simulink model "sampleModel145"  (R2021b)
settings: Solver=VariableStepAuto  StartTime=0.0  StopTime=10.0  RelTol=1e-3
libraries: simulink x1
settings Model: Creator=user  LastModifiedBy=user

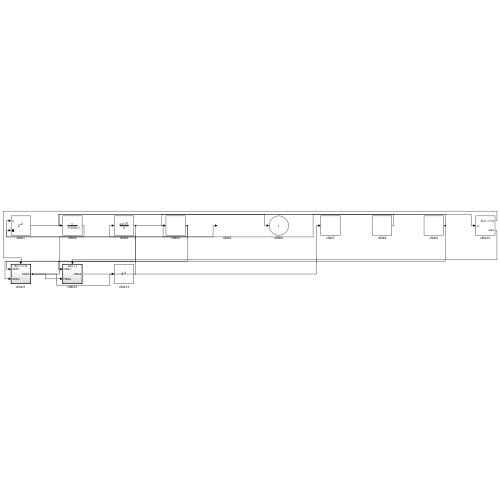
[thumbnail: Simulink's stored preview of the top-level diagram]
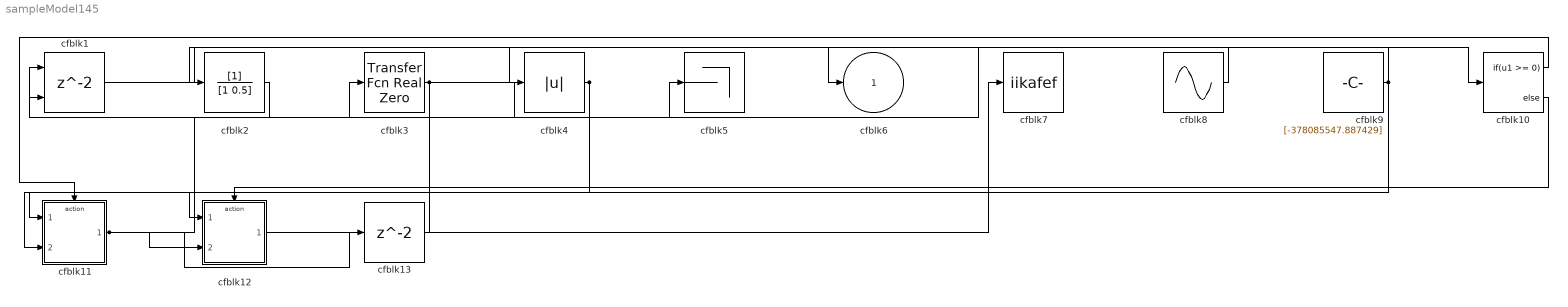
== system sampleModel145 ==
  cfblk1 : Delay  ShowEnablePort=on  SampleTime=1
      settings: InputPortMap=u0,e6
  cfblk10 : If  IfExpression=u1 >= 0  SampleTime=1
  cfblk11 : Subsystem  TreatAsAtomicUnit=on
  cfblk12 : Subsystem  TreatAsAtomicUnit=on
  cfblk13 : Delay  SampleTime=1
  cfblk2 : DiscreteFilter  SampleTime=1
  cfblk3 : simulink/Discrete/Transfer Fcn Real Zero  ZeroZ=0.75  ICPrevInput=0.0  DoSatur=off
      settings: SourceProductBaseCode=SL
  cfblk4 : Abs
  cfblk5 : Terminator
  cfblk7 : ToWorkspace  VariableName=iikafef  SaveFormat=Timeseries  SampleTime=-1
  cfblk8 : Sin  Amplitude=[-440683838.246815]  Bias=[450230892.144904]  SampleTime=0
  cfblk9 : Constant  Value=[-378085547.887429]  SampleTime=1
  cfblk6 : Outport
  wires:
  cfblk12/1(cfblk2) -> cfblk7/1
  cfblk1/1 -> cfblk6/1
  cfblk3/1 -> cfblk10/1, cfblk12/1(cfblk1)
  cfblk2/1 -> cfblk1/1
  cfblk11/1(cfblk2) -> cfblk5/1, cfblk12/2(cfblk4), cfblk13/1
  cfblk4/1 -> cfblk1/2, cfblk11/2(cfblk4)
  cfblk8/1 -> cfblk4/1
  cfblk9/1 -> cfblk2/1, cfblk11/1(cfblk1)
  cfblk10/1 -> cfblk11/Action
  cfblk10/2 -> cfblk12/Action
  cfblk13/1 -> cfblk3/1

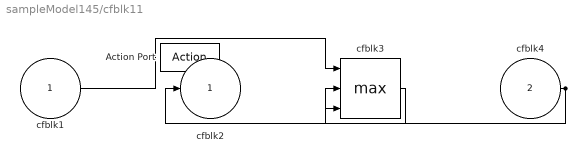
== system sampleModel145/cfblk11 ==
  cfblk1 : Inport
  cfblk4 : Inport  Port=2
  Action Port : ActionPort  ActionPortLabel=if(u1 >= 0)
  cfblk3 : MinMax  Function=max  Inputs=3
  cfblk2 : Outport
  wires:
  cfblk3/1 -> cfblk2/1
  cfblk1/1 -> cfblk3/1
  cfblk4/1 -> cfblk3/2, cfblk3/3

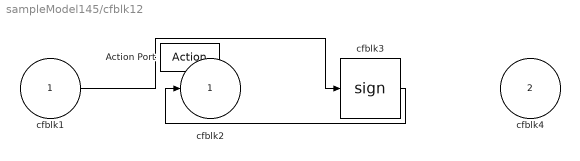
== system sampleModel145/cfblk12 ==
  cfblk1 : Inport
  cfblk4 : Inport  Port=2
  Action Port : ActionPort  ActionPortLabel=else
  cfblk3 : Signum
  cfblk2 : Outport
  wires:
  cfblk3/1 -> cfblk2/1
  cfblk1/1 -> cfblk3/1
